simulink model "vexarmcortex_BEST_SimBot_Dashboard"  (R2019a)
settings: Solver=FixedStepAuto  StartTime=0.0  StopTime=inf  RelTol=1e-3  EnableMultiTasking=on
libraries: vexarmcortexlib x13, simulink x1
settings Model: SimulationMode=external  ExtModeTrigDuration=25  Creator=The MathWorks, Inc.  LastModifiedBy=josea
settings DataIOCC: ReturnWorkspaceOutputs=off
settings OptimizationCC: MaxStackSize=64
settings DebuggingCC: ParameterTunabilityLossMsg=error  ArithmeticOperatorsInVariantConditions=warning
settings HardwareCC: ProdBitPerPointer=32  ProdBitPerSizeT=32  ProdBitPerPtrDiffT=32  ProdLargestAtomicInteger=Long  ProdLargestAtomicFloat=Double  ProdWordSize=32  ProdHWDeviceType=ARM Compatible->ARM Cortex  UseEmbeddedCoderFeatures=off
settings SFSimCC: SimUseLocalCustomCode=off
settings RTWCC: SystemTargetFile=ert.tlc  HardwareBoard=ARM Cortex-based VEX Microcontroller  TLCOptions="-aInlineSetEventsForThisBaseRateFcn=TLC_FALSE -aSuppressMultiTaskScheduler=TLC_FALSE  -aRateBasedStepFcn=0"  TemplateMakefile=ert_default_tmf  RTWUseLocalCustomCode=off  Toolchain=GNU Tools for VEX ARM Cortex
settings CodeAppCC: ForceParamTrailComments=on  OperatorAnnotations=on  StateflowObjectComments=on  MATLABSourceComments=on
settings ERTTargetCC: ERTCustomFileBanners=off  SupportContinuousTime=on  SupportNonInlinedSFcns=on  RemoveResetFunc=off  ModelStepFunctionPrototypeControlCompliant=off

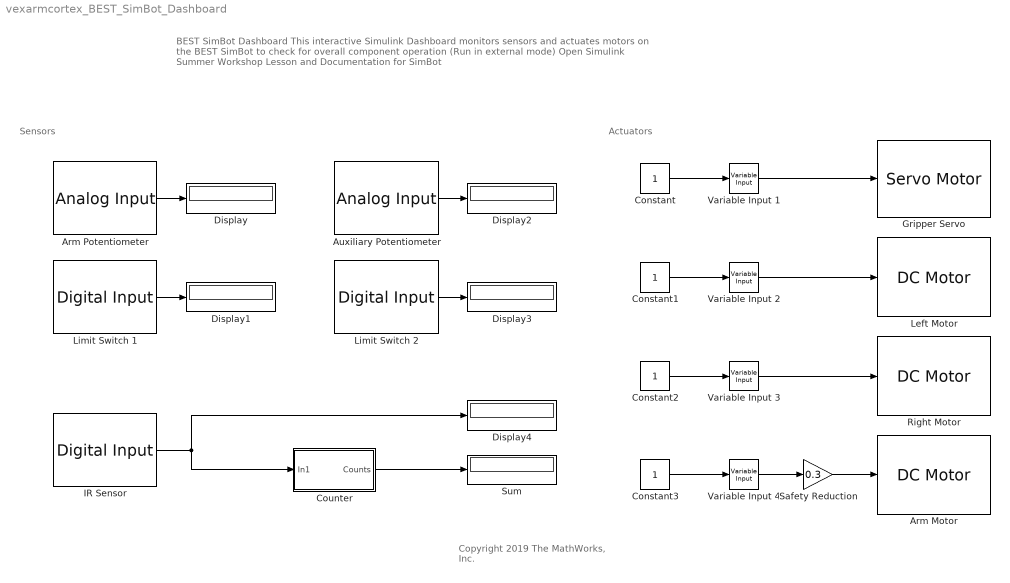
== system vexarmcortex_BEST_SimBot_Dashboard ==
  note: Actuators
  note: Sensors
  note: BEST SimBot Dashboard
      | This interactive Simulink Dashboard monitors sensors and actuates motors
      | on the BEST SimBot to check for overall component operation (Run in external mode)
      | Open Simulink Summer Workshop Lesson and Documentation for SimBot
  note: Copyright 2019 The MathWorks, Inc.
  Arm Motor : vexarmcortexlib/Actuators/DC Motor  motor=4  scaleFactor=1/13.5  SimulationOut=off
      settings: SourceProductName=Simulink Coder Support Package for ARM Cortex-based VEX Microcontroller  SourceProductBaseCode=EC_VEX_MICRO
  Arm Potentiometer : vexarmcortexlib/Sensors/Analog Input  inChan=1  SimulationIn=off  SampleTime=0.05
      settings: SourceProductName=Simulink Coder Support Package for ARM Cortex-based VEX Microcontroller  SourceProductBaseCode=EC_VEX_MICRO
  Auxiliary Potentiometer : vexarmcortexlib/Sensors/Analog Input  inChan=2  SimulationIn=off  SampleTime=0.05
      settings: SourceProductName=Simulink Coder Support Package for ARM Cortex-based VEX Microcontroller  SourceProductBaseCode=EC_VEX_MICRO
  Constant{,1..3} (4 alike) : Constant
  Counter : Subsystem
  Display{,1..4} (5 alike) : Display
  Gripper Servo : vexarmcortexlib/Actuators/Servo Motor  motor=2  scaleFactor=60/127  SimulationOut=off
      settings: SourceProductName=Simulink Coder Support Package for ARM Cortex-based VEX Microcontroller  SourceProductBaseCode=EC_VEX_MICRO
  IR Sensor : vexarmcortexlib/Sensors/Digital Input  inChan=3  SimulationIn=off  SampleTime=0.05
      settings: SourceProductName=Simulink Coder Support Package for ARM Cortex-based VEX Microcontroller  SourceProductBaseCode=EC_VEX_MICRO
  Left Motor : vexarmcortexlib/Actuators/DC Motor  motor=5  scaleFactor=1/13.5  SimulationOut=off
      settings: SourceProductName=Simulink Coder Support Package for ARM Cortex-based VEX Microcontroller  SourceProductBaseCode=EC_VEX_MICRO
  Limit Switch 1 : vexarmcortexlib/Sensors/Digital Input  inChan=1  SimulationIn=off  SampleTime=0.05
      settings: SourceProductName=Simulink Coder Support Package for ARM Cortex-based VEX Microcontroller  SourceProductBaseCode=EC_VEX_MICRO
  Limit Switch 2 : vexarmcortexlib/Sensors/Digital Input  inChan=2  SimulationIn=off  SampleTime=0.05
      settings: SourceProductName=Simulink Coder Support Package for ARM Cortex-based VEX Microcontroller  SourceProductBaseCode=EC_VEX_MICRO
  Right Motor : vexarmcortexlib/Actuators/DC Motor  motor=3  scaleFactor=1/13.5  SimulationOut=off
      settings: SourceProductName=Simulink Coder Support Package for ARM Cortex-based VEX Microcontroller  SourceProductBaseCode=EC_VEX_MICRO
  Safety Reduction : Gain  Gain=0.3
  Sum : Display
  Variable Input {1..4} (4 alike) : vexarmcortexlib/Utilities/Variable Input  low=-127  gain=0  high=127
      settings: SourceProductName=Simulink Coder Support Package for ARM Cortex-based VEX Microcontroller  SourceProductBaseCode=EC_VEX_MICRO
  wires:
  Arm Potentiometer/1 -> Display/1
  Limit Switch 1/1 -> Display1/1
  Auxiliary Potentiometer/1 -> Display2/1
  Limit Switch 2/1 -> Display3/1
  Variable Input 1/1 -> Gripper Servo/1
  Constant/1 -> Variable Input 1/1
  IR Sensor/1 -> Counter/1(In1), Display4/1
  Counter/1(Counts) -> Sum/1
  Constant1/1 -> Variable Input 2/1
  Constant2/1 -> Variable Input 3/1
  Variable Input 2/1 -> Left Motor/1
  Variable Input 3/1 -> Right Motor/1
  Variable Input 4/1 -> Safety Reduction/1
  Constant3/1 -> Variable Input 4/1
  Safety Reduction/1 -> Arm Motor/1

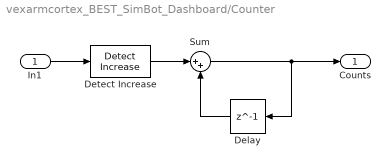
== system vexarmcortex_BEST_SimBot_Dashboard/Counter ==
  In1 : Inport
  Delay : Delay  DelayLength=1
  Detect Increase : simulink/Logic and Bit Operations/Detect Increase  vinit=0.0  OutDataTypeStr=uint8
  Sum : Sum  Inputs=|++
  Counts : Outport
  wires:
  In1/1 -> Detect Increase/1
  Detect Increase/1 -> Sum/1
  Sum/1 -> Delay/1, Counts/1
  Delay/1 -> Sum/2
